simulink model "hw2_eserc_4_simulink"  (R2023b)
settings: Solver=VariableStepAuto  StartTime=0.0  StopTime=10.0  RelTol=1e-3
undefined symbols (not defined in the file or in its folder): b, k1, k2
libraries: robotmobilelib x1
settings Model: Creator=ANDREA  LastModifiedBy=lalla

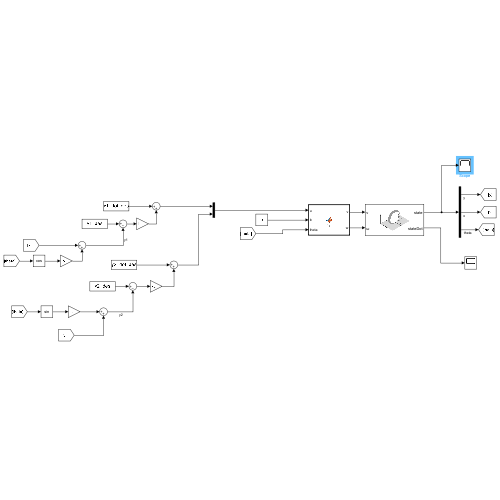
[thumbnail: Simulink's stored preview of the top-level diagram]
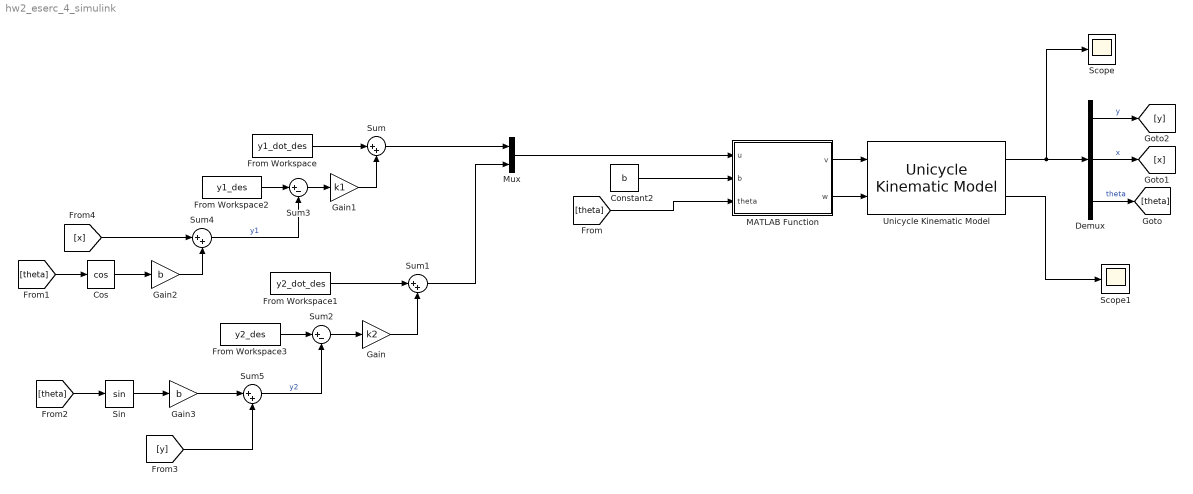
== system hw2_eserc_4_simulink ==
  Constant2 : Constant  Value=b
  Cos : Trigonometry  Operator=cos
  Demux : Demux  Outputs=3
  From Workspace : FromWorkspace  VariableName=y1_dot_des
  From Workspace1 : FromWorkspace  VariableName=y2_dot_des
  From Workspace2 : FromWorkspace  VariableName=y1_des
  From Workspace3 : FromWorkspace  VariableName=y2_des
  Gain : Gain  Gain=k2
  Gain1 : Gain  Gain=k1
  Gain2 : Gain  Gain=b
  Gain3 : Gain  Gain=b
  MATLAB Function : MATLAB Function  TreatAsAtomicUnit=on
  Mux : Mux  Inputs=2
  Scope : Scope
  Scope1 : Scope
  Sin : Trigonometry
  Sum{,1,4..5} (4 alike) : Sum  Inputs=|++
  Sum2 : Sum  Inputs=|+-
  Sum3 : Sum  Inputs=|+-
  Unicycle Kinematic Model : robotmobilelib/Unicycle Kinematic Model  VehicleInputs=Vehicle Speed & Heading Angular Velocity  WheelRadius=0.1  WheelSpeedRange=[-Inf Inf]  InitialState=[0; 0; 0]  SimulateUsing=Interpreted execution
  wires:
  Unicycle Kinematic Model/1 -> Demux/1, Scope/1
  Unicycle Kinematic Model/2 -> Scope1/1
  From Workspace/1 -> Sum/1
  From Workspace1/1 -> Sum1/1
  Gain/1 -> Sum1/2
  Gain1/1 -> Sum/2
  Sum3/1 -> Gain1/1
  Sum2/1 -> Gain/1
  From Workspace3/1 -> Sum2/1
  From Workspace2/1 -> Sum3/1
  Sum4/1 -> Sum3/2  "y1"
  Sum5/1 -> Sum2/2  "y2"
  Constant2/1 -> MATLAB Function/2(b)
  Cos/1 -> Gain2/1
  Sin/1 -> Gain3/1
  Demux/3 -> [theta]  "theta"
  [theta] -> MATLAB Function/3(theta)
  [theta] -> Cos/1
  [theta] -> Sin/1
  Gain2/1 -> Sum4/2
  Sum/1 -> Mux/1
  Sum1/1 -> Mux/2
  Mux/1 -> MATLAB Function/1(u)
  MATLAB Function/1(v) -> Unicycle Kinematic Model/1
  MATLAB Function/2(w) -> Unicycle Kinematic Model/2
  Demux/1 -> [y]  "y"
  Demux/2 -> [x]  "x"
  [x] -> Sum4/1
  Gain3/1 -> Sum5/1
  [y] -> Sum5/2

== matlab function hw2_eserc_4_simulink/MATLAB Function ==
  data: u input; b input; theta input; v output; w output
function [v,w] = fcn(u, b, theta)
T = [cos(theta) -b*sin(theta);
     sin(theta) b*cos(theta)];
sol = inv(T)*u;
v = sol(1,:);
w = sol(2,:);
